simulink model "Test_SimFEAdapter"  (Simulink 7.5)
settings: Solver=FixedStepDiscrete  StartTime=0.0  StopTime=inf  FixedStep=samplePeriod  RelTol=1e-3  AbsTol=1e-6
PreLoadFcn:
  | initializeSimulation
InitFcn:
  | clear('all');
  | initializeSimulation;
values from neighbouring files (symbols this model uses):
  damperA = 0    [initializeSimulation.m]
  damperB = 0    [initializeSimulation.m]
  damperC = 0    [initializeSimulation.m]
  damperCanon = 1    [initializeSimulation.m]
  flowCanon = 3.85    [initializeSimulation.m]
  forceCanon = 1    [initializeSimulation.m]
  frictionA = 0    [initializeSimulation.m]
  frictionB = 0    [initializeSimulation.m]
  frictionC = 0    [initializeSimulation.m]
  gasConstant = 1.8    [initializeSimulation.m]
  lengthCanon = 1    [initializeSimulation.m]
  massA = 4.2    [initializeSimulation.m]
  massB = 2.5    [initializeSimulation.m]
  massC = 2.5    [initializeSimulation.m]
  massCanon = 0.002588    [initializeSimulation.m]
  maxDisplA = (stroke2A + endLength2A) * lengthCanon    (= 22)    [initializeSimulation.m]
  maxDisplB = (stroke2B + endLength2B) * lengthCanon    (= 42)    [initializeSimulation.m]
  maxDisplC = (stroke2C + endLength2C) * lengthCanon    (= 72)    [initializeSimulation.m]
  maxOilVolume = volume * (1 - (precharge/supplyPress)^(1/gasConstant))    (= 10.5071802963)    [initializeSimulation.m]
  maxVelocA = (maxFlowA * flowCanon / (area1A * areaCanon)) / velocCanon    [initializeSimulation.m]
  maxVelocB = (maxFlowB * flowCanon / (area1B * areaCanon)) / velocCanon    [initializeSimulation.m]
  maxVelocC = (maxFlowC * flowCanon / (area1C * areaCanon)) / velocCanon    [initializeSimulation.m]
  minDisplA = -(stroke1A + endLength1A) * lengthCanon    (= -22)    [initializeSimulation.m]
  minDisplB = -(stroke1B + endLength1B) * lengthCanon    (= -42)    [initializeSimulation.m]
  minDisplC = -(stroke1C + endLength1C) * lengthCanon    (= -72)    [initializeSimulation.m]
  minVelocA = -(maxFlowA * flowCanon / (area2A * areaCanon)) / velocCanon    [initializeSimulation.m]
  minVelocB = -(maxFlowB * flowCanon / (area2B * areaCanon)) / velocCanon    [initializeSimulation.m]
  minVelocC = -(maxFlowC * flowCanon / (area2C * areaCanon)) / velocCanon    [initializeSimulation.m]
  nAct = 8    [initializeSimulation.m]
  nAdcU = 12    [initializeSimulation.m]
  nDinp = 4    [initializeSimulation.m]
  nDout = 4    [initializeSimulation.m]
  nDucU = 8    [initializeSimulation.m]
  nEncU = 2    [initializeSimulation.m]
  precharge = 1000    [initializeSimulation.m]
  pumpFlow = 1e10    (= 10000000000)    [initializeSimulation.m]
  returnPress = 50    [initializeSimulation.m]
  staticForceA = 0    [initializeSimulation.m]
  staticForceB = 0    [initializeSimulation.m]
  staticForceC = 0    [initializeSimulation.m]
  supplyPress = 3000    [initializeSimulation.m]
  velocCanon = 1    [initializeSimulation.m]
  volume = accumVolume * accumNumber    (= 23)    [initializeSimulation.m]
  volumeCanon = 231    [initializeSimulation.m]
  yieldDisplA = 0.1    [initializeSimulation.m]
  yieldDisplB = 0.1    [initializeSimulation.m]
  yieldDisplC = 0.1    [initializeSimulation.m]
undefined symbols (not defined in the file or in its folder): DiscIntNeverNeededParam
(part 2 of 3)

== system Test_SimFEAdapter/model/ActuatorPayloadMdl/static channel #1/actuator/valve  model ==
  note: Note: "1" and "2" denote actuator
      | cylinders on either side of the
      | actuator piston.  With positive
      | valve drive, oil is ported into
      | cylinder 1, resulting in positive
      | displacement.
  note: Auxiliary diagnostic output vector:
      | 1:   valve opening
      | 2:   C1 pressure
      | 3:   C2 pressure
      | 4:   delta pressure
      | 5:   force
      | 6:   velocity
      | 7:   C1 flow
      | 8:   C2 flow
      | 9:   total flow
      | 10: kinematic flow
      | 11: compressibility flow
      | 12: leakage flow
  note: Parameter vector:
      | 1:   oil bulk modulus (force/displ^2)
      | 2:   servovalve delay (sec)
      | 3:   servovalve overlap
      | 4:   rated pressure (force/displ^2)
      | 5:   rated flow at rated pressure (displ^3/sec)
      | 6:   nominal flow at rated pressure (displ^3/sec)
      | 7:   actuator piston area 1 (displ^2)
      | 8:   actuator piston area 2 (displ^2)
      | 9:   actuator usable stroke 1 (displ)
      | 10: actuator usable stroke 2 (displ)
      | 11: actuator end cushion length 1 (displ)
      | 12: actuator end cushion length 2 (displ)
      | 13: actuator parasitic damping factor
      | 14: cross-chamber leakage factor (flow/press)
      | 15: ratio port openings according to area
      | 16: sample period (sec)
      |
      | Conversion factors used for converting
      | signals from external (user) to internal
      | (canonical) units:
      |
      | 17: displacement
      | 18: velocity
      | 19: force
      | 20: pressure
      | 21: flow
  cmd : Inport  OutDataType=sfix(16)  OutScaling=2^0
  displ : Inport  Port=2  OutDataType=sfix(16)  OutScaling=2^0
  veloc : Inport  Port=3  OutDataType=sfix(16)  OutScaling=2^0
  spl press : Inport  Port=4  OutDataType=sfix(16)  OutScaling=2^0
  rtn press : Inport  Port=5  OutDataType=sfix(16)  OutScaling=2^0
  abs : Abs  SaturateOnIntegerOverflow=on
  actuator : S-Function  FunctionName=actuator  Parameters=actParamsC  EnableBusSupport=off
  total flow sel : Selector  InputPortWidth=12  IndexOptions=Index vector (dialog)  Indices=9  OutputSizes=1
  force : Outport  OutDataType=sfix(16)  OutScaling=2^0
  flow : Outport  Port=2  OutDataType=sfix(16)  OutScaling=2^0
  wires:
  veloc/1 -> actuator/3
  displ/1 -> actuator/2
  actuator/1 -> force/1
  cmd/1 -> actuator/1
  rtn press/1 -> actuator/5
  spl press/1 -> actuator/4
  total flow sel/1 -> abs/1
  actuator/2 -> total flow sel/1
  abs/1 -> flow/1

== system Test_SimFEAdapter/model/ActuatorPayloadMdl/static channel #1/payload ==
  force : Inport  OutDataType=sfix(16)  OutScaling=2^0
  Sum : Sum  Inputs=+----  OutDataType=sfix(16)  OutScaling=2^0  SaturateOnIntegerOverflow=on  InputSameDT=on  OutDataTypeStr=Inherit: Same as first input
  damper : Gain  Gain=damperC*damperCanon  ParameterDataType=sfix(16)  ParameterScaling=2^0  OutDataType=sfix(16)  OutScaling=2^0  SaturateOnIntegerOverflow=on  OutDataTypeStr=Inherit: Same as input  ParamDataTypeStr=Inherit: Same as input
  div : Product  Inputs=*/  OutDataType=sfix(16)  OutScaling=2^0  SaturateOnIntegerOverflow=on  InputSameDT=on  OutDataTypeStr=Inherit: Same as first input
  double integrator : Subsystem
  friction : Subsystem  mask{friction=frictionC*forceCanon, yieldDispl=yieldDisplC*lengthCanon, hysteresis=0}
      mask prompts: friction "Sliding friction"; yieldDispl "Equiv. yield displacement (in)"; hysteresis "Hysteresis constant"
  mass : Constant  Value=massC*massCanon  OutDataType=sfix(16)  OutScaling=2^0
  static force : Constant  Value=staticForceC*forceCanon  OutDataType=sfix(16)  OutScaling=2^0
  term1 : Terminator
  unit dly : UnitDelay  SampleTime=-1
  unit dly1 : UnitDelay  SampleTime=-1
  veloc units : Gain  Gain=1/velocCanon  ParameterDataType=sfix(16)  ParameterScaling=2^0  OutDataType=sfix(16)  OutScaling=2^0  SaturateOnIntegerOverflow=on  OutDataTypeStr=Inherit: Same as input  ParamDataTypeStr=Inherit: Same as input
  displ : Outport  OutDataType=sfix(16)  OutScaling=2^0
  veloc : Outport  Port=2  OutDataType=sfix(16)  OutScaling=2^0
  tag scope: ch5a=global
  wires:
  friction/1(force) -> Sum/2  "friction force"
  veloc units/1 -> veloc/1
  Sum/1 -> div/1  "inertial force"
  force/1 -> Sum/1  "total force"
  mass/1 -> div/2
  double integrator/3(acc) -> term1/1
  div/1 -> double integrator/1(accel)
  double integrator/1(displ) -> displ/1, unit dly/1
  double integrator/2(veloc) -> veloc units/1, friction/1(veloc), unit dly1/1
  static force/1 -> Sum/5  "static force"
  damper/1 -> Sum/4  "damper force"
  unit dly1/1 -> damper/1
  [ch5b] -> Sum/3  "spring force"
  unit dly/1 -> [ch5a]

== system Test_SimFEAdapter/model/ActuatorPayloadMdl/static channel #2/actuator/valve  model ==
  note: Auxiliary diagnostic output vector:
      | 1:   valve opening
      | 2:   C1 pressure
      | 3:   C2 pressure
      | 4:   delta pressure
      | 5:   force
      | 6:   velocity
      | 7:   C1 flow
      | 8:   C2 flow
      | 9:   total flow
      | 10: kinematic flow
      | 11: compressibility flow
      | 12: leakage flow
  note: Note: "1" and "2" denote actuator
      | cylinders on either side of the
      | actuator piston.  With positive
      | valve drive, oil is ported into
      | cylinder 1, resulting in positive
      | displacement.
  note: Parameter vector:
      | 1:   oil bulk modulus (force/displ^2)
      | 2:   servovalve delay (sec)
      | 3:   servovalve overlap
      | 4:   rated pressure (force/displ^2)
      | 5:   rated flow at rated pressure (displ^3/sec)
      | 6:   nominal flow at rated pressure (displ^3/sec)
      | 7:   actuator piston area 1 (displ^2)
      | 8:   actuator piston area 2 (displ^2)
      | 9:   actuator usable stroke 1 (displ)
      | 10: actuator usable stroke 2 (displ)
      | 11: actuator end cushion length 1 (displ)
      | 12: actuator end cushion length 2 (displ)
      | 13: actuator parasitic damping factor
      | 14: cross-chamber leakage factor (flow/press)
      | 15: ratio port openings according to area
      | 16: sample period (sec)
      |
      | Conversion factors used for converting
      | signals from external (user) to internal
      | (canonical) units:
      |
      | 17: displacement
      | 18: velocity
      | 19: force
      | 20: pressure
      | 21: flow
  cmd : Inport  OutDataType=sfix(16)  OutScaling=2^0
  displ : Inport  Port=2  OutDataType=sfix(16)  OutScaling=2^0
  veloc : Inport  Port=3  OutDataType=sfix(16)  OutScaling=2^0
  spl press : Inport  Port=4  OutDataType=sfix(16)  OutScaling=2^0
  rtn press : Inport  Port=5  OutDataType=sfix(16)  OutScaling=2^0
  abs : Abs  SaturateOnIntegerOverflow=on
  actuator : S-Function  FunctionName=actuator  Parameters=actParamsC  EnableBusSupport=off
  total flow sel : Selector  InputPortWidth=12  IndexOptions=Index vector (dialog)  Indices=9  OutputSizes=1
  force : Outport  OutDataType=sfix(16)  OutScaling=2^0
  flow : Outport  Port=2  OutDataType=sfix(16)  OutScaling=2^0
  wires:
  abs/1 -> flow/1
  actuator/2 -> total flow sel/1
  total flow sel/1 -> abs/1
  spl press/1 -> actuator/4
  rtn press/1 -> actuator/5
  cmd/1 -> actuator/1
  actuator/1 -> force/1
  displ/1 -> actuator/2
  veloc/1 -> actuator/3

== system Test_SimFEAdapter/model/ActuatorPayloadMdl/static channel #2/payload ==
  force : Inport  OutDataType=sfix(16)  OutScaling=2^0
  Sum : Sum  Inputs=+----  OutDataType=sfix(16)  OutScaling=2^0  SaturateOnIntegerOverflow=on  InputSameDT=on  OutDataTypeStr=Inherit: Same as first input
  damper : Gain  Gain=damperC*damperCanon  ParameterDataType=sfix(16)  ParameterScaling=2^0  OutDataType=sfix(16)  OutScaling=2^0  SaturateOnIntegerOverflow=on  OutDataTypeStr=Inherit: Same as input  ParamDataTypeStr=Inherit: Same as input
  div : Product  Inputs=*/  OutDataType=sfix(16)  OutScaling=2^0  SaturateOnIntegerOverflow=on  InputSameDT=on  OutDataTypeStr=Inherit: Same as first input
  double integrator : Subsystem
  friction : Subsystem  mask{friction=frictionC*forceCanon, yieldDispl=yieldDisplC*lengthCanon, hysteresis=0}
      mask prompts: friction "Sliding friction"; yieldDispl "Equiv. yield displacement (in)"; hysteresis "Hysteresis constant"
  mass : Constant  Value=massC*massCanon  OutDataType=sfix(16)  OutScaling=2^0
  static force : Constant  Value=staticForceC*forceCanon  OutDataType=sfix(16)  OutScaling=2^0
  term1 : Terminator
  unit dly : UnitDelay  SampleTime=-1
  unit dly1 : UnitDelay  SampleTime=-1
  veloc units : Gain  Gain=1/velocCanon  ParameterDataType=sfix(16)  ParameterScaling=2^0  OutDataType=sfix(16)  OutScaling=2^0  SaturateOnIntegerOverflow=on  OutDataTypeStr=Inherit: Same as input  ParamDataTypeStr=Inherit: Same as input
  displ : Outport  OutDataType=sfix(16)  OutScaling=2^0
  veloc : Outport  Port=2  OutDataType=sfix(16)  OutScaling=2^0
  tag scope: ch6a=global
  wires:
  friction/1(force) -> Sum/2  "friction force"
  veloc units/1 -> veloc/1
  Sum/1 -> div/1  "inertial force"
  force/1 -> Sum/1  "total force"
  mass/1 -> div/2
  double integrator/3(acc) -> term1/1
  div/1 -> double integrator/1(accel)
  double integrator/1(displ) -> displ/1, unit dly/1
  double integrator/2(veloc) -> veloc units/1, friction/1(veloc), unit dly1/1
  static force/1 -> Sum/5  "static force"
  damper/1 -> Sum/4  "damper force"
  unit dly1/1 -> damper/1
  [ch6b] -> Sum/3  "spring force"
  unit dly/1 -> [ch6a]

== system Test_SimFEAdapter/model/ActuatorPayloadMdl/static channel #3/actuator/valve  model ==
  note: Note: "1" and "2" denote actuator
      | cylinders on either side of the
      | actuator piston.  With positive
      | valve drive, oil is ported into
      | cylinder 1, resulting in positive
      | displacement.
  note: Auxiliary diagnostic output vector:
      | 1:   valve opening
      | 2:   C1 pressure
      | 3:   C2 pressure
      | 4:   delta pressure
      | 5:   force
      | 6:   velocity
      | 7:   C1 flow
      | 8:   C2 flow
      | 9:   total flow
      | 10: kinematic flow
      | 11: compressibility flow
      | 12: leakage flow
  note: Parameter vector:
      | 1:   oil bulk modulus (force/displ^2)
      | 2:   servovalve delay (sec)
      | 3:   servovalve overlap
      | 4:   rated pressure (force/displ^2)
      | 5:   rated flow at rated pressure (displ^3/sec)
      | 6:   nominal flow at rated pressure (displ^3/sec)
      | 7:   actuator piston area 1 (displ^2)
      | 8:   actuator piston area 2 (displ^2)
      | 9:   actuator usable stroke 1 (displ)
      | 10: actuator usable stroke 2 (displ)
      | 11: actuator end cushion length 1 (displ)
      | 12: actuator end cushion length 2 (displ)
      | 13: actuator parasitic damping factor
      | 14: cross-chamber leakage factor (flow/press)
      | 15: ratio port openings according to area
      | 16: sample period (sec)
      |
      | Conversion factors used for converting
      | signals from external (user) to internal
      | (canonical) units:
      |
      | 17: displacement
      | 18: velocity
      | 19: force
      | 20: pressure
      | 21: flow
  cmd : Inport  OutDataType=sfix(16)  OutScaling=2^0
  displ : Inport  Port=2  OutDataType=sfix(16)  OutScaling=2^0
  veloc : Inport  Port=3  OutDataType=sfix(16)  OutScaling=2^0
  spl press : Inport  Port=4  OutDataType=sfix(16)  OutScaling=2^0
  rtn press : Inport  Port=5  OutDataType=sfix(16)  OutScaling=2^0
  abs : Abs  SaturateOnIntegerOverflow=on
  actuator : S-Function  FunctionName=actuator  Parameters=actParamsC  EnableBusSupport=off
  total flow sel : Selector  InputPortWidth=12  IndexOptions=Index vector (dialog)  Indices=9  OutputSizes=1
  force : Outport  OutDataType=sfix(16)  OutScaling=2^0
  flow : Outport  Port=2  OutDataType=sfix(16)  OutScaling=2^0
  wires:
  veloc/1 -> actuator/3
  displ/1 -> actuator/2
  actuator/1 -> force/1
  cmd/1 -> actuator/1
  rtn press/1 -> actuator/5
  spl press/1 -> actuator/4
  total flow sel/1 -> abs/1
  actuator/2 -> total flow sel/1
  abs/1 -> flow/1

== system Test_SimFEAdapter/model/ActuatorPayloadMdl/static channel #3/payload ==
  force : Inport  OutDataType=sfix(16)  OutScaling=2^0
  Sum : Sum  Inputs=+----  OutDataType=sfix(16)  OutScaling=2^0  SaturateOnIntegerOverflow=on  InputSameDT=on  OutDataTypeStr=Inherit: Same as first input
  damper : Gain  Gain=damperC*damperCanon  ParameterDataType=sfix(16)  ParameterScaling=2^0  OutDataType=sfix(16)  OutScaling=2^0  SaturateOnIntegerOverflow=on  OutDataTypeStr=Inherit: Same as input  ParamDataTypeStr=Inherit: Same as input
  div : Product  Inputs=*/  OutDataType=sfix(16)  OutScaling=2^0  SaturateOnIntegerOverflow=on  InputSameDT=on  OutDataTypeStr=Inherit: Same as first input
  double integrator : Subsystem
  friction : Subsystem  mask{friction=frictionC*forceCanon, yieldDispl=yieldDisplC*lengthCanon, hysteresis=0}
      mask prompts: friction "Sliding friction"; yieldDispl "Equiv. yield displacement (in)"; hysteresis "Hysteresis constant"
  mass : Constant  Value=massC*massCanon  OutDataType=sfix(16)  OutScaling=2^0
  static force : Constant  Value=staticForceC*forceCanon  OutDataType=sfix(16)  OutScaling=2^0
  term1 : Terminator
  unit dly : UnitDelay  SampleTime=-1
  unit dly1 : UnitDelay  SampleTime=-1
  veloc units : Gain  Gain=1/velocCanon  ParameterDataType=sfix(16)  ParameterScaling=2^0  OutDataType=sfix(16)  OutScaling=2^0  SaturateOnIntegerOverflow=on  OutDataTypeStr=Inherit: Same as input  ParamDataTypeStr=Inherit: Same as input
  displ : Outport  OutDataType=sfix(16)  OutScaling=2^0
  veloc : Outport  Port=2  OutDataType=sfix(16)  OutScaling=2^0
  tag scope: ch7a=global
  wires:
  friction/1(force) -> Sum/2  "friction force"
  veloc units/1 -> veloc/1
  Sum/1 -> div/1  "inertial force"
  force/1 -> Sum/1  "total force"
  mass/1 -> div/2
  double integrator/3(acc) -> term1/1
  div/1 -> double integrator/1(accel)
  double integrator/1(displ) -> displ/1, unit dly/1
  double integrator/2(veloc) -> veloc units/1, friction/1(veloc), unit dly1/1
  static force/1 -> Sum/5  "static force"
  damper/1 -> Sum/4  "damper force"
  unit dly1/1 -> damper/1
  [ch7b] -> Sum/3  "spring force"
  unit dly/1 -> [ch7a]

== system Test_SimFEAdapter/model/ActuatorPayloadMdl/static channel #4/actuator/valve  model ==
  note: Auxiliary diagnostic output vector:
      | 1:   valve opening
      | 2:   C1 pressure
      | 3:   C2 pressure
      | 4:   delta pressure
      | 5:   force
      | 6:   velocity
      | 7:   C1 flow
      | 8:   C2 flow
      | 9:   total flow
      | 10: kinematic flow
      | 11: compressibility flow
      | 12: leakage flow
  note: Note: "1" and "2" denote actuator
      | cylinders on either side of the
      | actuator piston.  With positive
      | valve drive, oil is ported into
      | cylinder 1, resulting in positive
      | displacement.
  note: Parameter vector:
      | 1:   oil bulk modulus (force/displ^2)
      | 2:   servovalve delay (sec)
      | 3:   servovalve overlap
      | 4:   rated pressure (force/displ^2)
      | 5:   rated flow at rated pressure (displ^3/sec)
      | 6:   nominal flow at rated pressure (displ^3/sec)
      | 7:   actuator piston area 1 (displ^2)
      | 8:   actuator piston area 2 (displ^2)
      | 9:   actuator usable stroke 1 (displ)
      | 10: actuator usable stroke 2 (displ)
      | 11: actuator end cushion length 1 (displ)
      | 12: actuator end cushion length 2 (displ)
      | 13: actuator parasitic damping factor
      | 14: cross-chamber leakage factor (flow/press)
      | 15: ratio port openings according to area
      | 16: sample period (sec)
      |
      | Conversion factors used for converting
      | signals from external (user) to internal
      | (canonical) units:
      |
      | 17: displacement
      | 18: velocity
      | 19: force
      | 20: pressure
      | 21: flow
  cmd : Inport  OutDataType=sfix(16)  OutScaling=2^0
  displ : Inport  Port=2  OutDataType=sfix(16)  OutScaling=2^0
  veloc : Inport  Port=3  OutDataType=sfix(16)  OutScaling=2^0
  spl press : Inport  Port=4  OutDataType=sfix(16)  OutScaling=2^0
  rtn press : Inport  Port=5  OutDataType=sfix(16)  OutScaling=2^0
  abs : Abs  SaturateOnIntegerOverflow=on
  actuator : S-Function  FunctionName=actuator  Parameters=actParamsC  EnableBusSupport=off
  total flow sel : Selector  InputPortWidth=12  IndexOptions=Index vector (dialog)  Indices=9  OutputSizes=1
  force : Outport  OutDataType=sfix(16)  OutScaling=2^0
  flow : Outport  Port=2  OutDataType=sfix(16)  OutScaling=2^0
  wires:
  abs/1 -> flow/1
  actuator/2 -> total flow sel/1
  total flow sel/1 -> abs/1
  spl press/1 -> actuator/4
  rtn press/1 -> actuator/5
  cmd/1 -> actuator/1
  actuator/1 -> force/1
  displ/1 -> actuator/2
  veloc/1 -> actuator/3

== system Test_SimFEAdapter/model/ActuatorPayloadMdl/static channel #4/payload ==
  force : Inport  OutDataType=sfix(16)  OutScaling=2^0
  Sum : Sum  Inputs=+----  OutDataType=sfix(16)  OutScaling=2^0  SaturateOnIntegerOverflow=on  InputSameDT=on  OutDataTypeStr=Inherit: Same as first input
  damper : Gain  Gain=damperC*damperCanon  ParameterDataType=sfix(16)  ParameterScaling=2^0  OutDataType=sfix(16)  OutScaling=2^0  SaturateOnIntegerOverflow=on  OutDataTypeStr=Inherit: Same as input  ParamDataTypeStr=Inherit: Same as input
  div : Product  Inputs=*/  OutDataType=sfix(16)  OutScaling=2^0  SaturateOnIntegerOverflow=on  InputSameDT=on  OutDataTypeStr=Inherit: Same as first input
  double integrator : Subsystem
  friction : Subsystem  mask{friction=frictionC*forceCanon, yieldDispl=yieldDisplC*lengthCanon, hysteresis=0}
      mask prompts: friction "Sliding friction"; yieldDispl "Equiv. yield displacement (in)"; hysteresis "Hysteresis constant"
  mass : Constant  Value=massC*massCanon  OutDataType=sfix(16)  OutScaling=2^0
  static force : Constant  Value=staticForceC*forceCanon  OutDataType=sfix(16)  OutScaling=2^0
  term1 : Terminator
  unit dly : UnitDelay  SampleTime=-1
  unit dly1 : UnitDelay  SampleTime=-1
  veloc units : Gain  Gain=1/velocCanon  ParameterDataType=sfix(16)  ParameterScaling=2^0  OutDataType=sfix(16)  OutScaling=2^0  SaturateOnIntegerOverflow=on  OutDataTypeStr=Inherit: Same as input  ParamDataTypeStr=Inherit: Same as input
  displ : Outport  OutDataType=sfix(16)  OutScaling=2^0
  veloc : Outport  Port=2  OutDataType=sfix(16)  OutScaling=2^0
  tag scope: ch8a=global
  wires:
  friction/1(force) -> Sum/2  "friction force"
  veloc units/1 -> veloc/1
  Sum/1 -> div/1  "inertial force"
  force/1 -> Sum/1  "total force"
  mass/1 -> div/2
  double integrator/3(acc) -> term1/1
  div/1 -> double integrator/1(accel)
  double integrator/1(displ) -> displ/1, unit dly/1
  double integrator/2(veloc) -> veloc units/1, friction/1(veloc), unit dly1/1
  static force/1 -> Sum/5  "static force"
  damper/1 -> Sum/4  "damper force"
  unit dly1/1 -> damper/1
  [ch8b] -> Sum/3  "spring force"
  unit dly/1 -> [ch8a]

== system Test_SimFEAdapter/model/ActuatorPayloadMdl/dynamic long channel #1/payload/double integrator ==
  accel : Inport
  displ gen : DiscreteIntegrator  IntegratorMethod=Integration: Backward Euler  SampleTime=-1  OutDataType=sfix(16)  OutScaling=2^0  LimitOutput=on  UpperSaturationLimit=maxDisplB  LowerSaturationLimit=minDisplB  ShowSaturationPort=on  ICPrevOutput=DiscIntNeverNeededParam  ICPrevScaledInput=DiscIntNeverNeededParam
  veloc gen : Subsystem  mask{maxVeloc=maxVelocB*velocCanon, minVeloc=minVelocB*velocCanon, maxDispl=maxDisplB, minDispl=minDisplB}
      mask prompts: maxVeloc "Max velocity"; minVeloc "Min velocity"; maxDispl "Max displacement"; minDispl "Min displacement"
  displ : Outport
  veloc : Outport  Port=2
  acc : Outport  Port=3
  wires:
  displ gen/2 -> veloc gen/3(reset)
  displ gen/1 -> displ/1, veloc gen/2(displ)
  veloc gen/1(veloc) -> displ gen/1, veloc/1
  accel/1 -> veloc gen/1(accel), acc/1

== system Test_SimFEAdapter/model/ActuatorPayloadMdl/dynamic long channel #1/payload/friction ==
  veloc : Inport  OutDataType=sfix(16)  OutScaling=2^0
  1-beta : Gain  Gain=1-hysteresis  ParameterDataType=sfix(16)  ParameterScaling=2^0  OutDataType=sfix(16)  OutScaling=2^0  SaturateOnIntegerOverflow=on  OutDataTypeStr=Inherit: Same as input  ParamDataTypeStr=Inherit: Same as input
  Sign : Signum
  Sum : Sum  Inputs=|++  OutDataType=sfix(16)  OutScaling=2^0  SaturateOnIntegerOverflow=on
  Sum1 : Sum  Inputs=|+-  OutDataType=sfix(16)  OutScaling=2^0  SaturateOnIntegerOverflow=on
  beta : Constant  Value=hysteresis  OutDataType=sfix(16)  OutScaling=2^0
  integrator : DiscreteIntegrator  SampleTime=-1  OutDataType=sfix(16)  OutScaling=2^0  LimitOutput=on  UpperSaturationLimit=1  LowerSaturationLimit=-1  ICPrevOutput=DiscIntNeverNeededParam  ICPrevScaledInput=DiscIntNeverNeededParam
  one : Constant  OutDataType=sfix(16)  OutScaling=2^0
  prod1 : Product  OutDataType=sfix(16)  OutScaling=2^0  SaturateOnIntegerOverflow=on  InputSameDT=on  OutDataTypeStr=Inherit: Same as first input
  prod2 : Product  OutDataType=sfix(16)  OutScaling=2^0  SaturateOnIntegerOverflow=on  InputSameDT=on  OutDataTypeStr=Inherit: Same as first input
  prod3 : Product  Inputs=3  OutDataType=sfix(16)  OutScaling=2^0  SaturateOnIntegerOverflow=on  InputSameDT=on  OutDataTypeStr=Inherit: Same as first input
  prod4 : Product  OutDataType=sfix(16)  OutScaling=2^0  SaturateOnIntegerOverflow=on  InputSameDT=on  OutDataTypeStr=Inherit: Same as first input
  sliding friction : Constant  Value=friction  OutDataType=sfix(16)  OutScaling=2^0
  y inv : Gain  Gain=1/max(eps, yieldDispl)  ParameterDataType=sfix(16)  ParameterScaling=2^0  OutDataType=sfix(16)  OutScaling=2^0  SaturateOnIntegerOverflow=on  OutDataTypeStr=Inherit: Same as input  ParamDataTypeStr=Inherit: Same as input
  force : Outport  OutDataType=sfix(16)  OutScaling=2^0
  wires:
  sliding friction/1 -> prod1/1
  prod1/1 -> force/1
  veloc/1 -> prod4/2, prod2/2
  prod4/1 -> Sign/1
  Sign/1 -> 1-beta/1
  1-beta/1 -> Sum/2
  beta/1 -> Sum/1
  Sum/1 -> prod3/3
  one/1 -> Sum1/1
  prod3/1 -> Sum1/2
  Sum1/1 -> prod2/1
  prod2/1 -> y inv/1
  y inv/1 -> integrator/1
  integrator/1 -> prod1/2, prod4/1, prod3/1, prod3/2  "zee"

== system Test_SimFEAdapter/model/ActuatorPayloadMdl/dynamic long channel #2/payload/double integrator ==
  accel : Inport
  displ gen : DiscreteIntegrator  IntegratorMethod=Integration: Backward Euler  SampleTime=-1  OutDataType=sfix(16)  OutScaling=2^0  LimitOutput=on  UpperSaturationLimit=maxDisplB  LowerSaturationLimit=minDisplB  ShowSaturationPort=on  ICPrevOutput=DiscIntNeverNeededParam  ICPrevScaledInput=DiscIntNeverNeededParam
  veloc gen : Subsystem  mask{maxVeloc=maxVelocB*velocCanon, minVeloc=minVelocB*velocCanon, maxDispl=maxDisplB, minDispl=minDisplB}
      mask prompts: maxVeloc "Max velocity"; minVeloc "Min velocity"; maxDispl "Max displacement"; minDispl "Min displacement"
  displ : Outport
  veloc : Outport  Port=2
  acc : Outport  Port=3
  wires:
  displ gen/2 -> veloc gen/3(reset)
  displ gen/1 -> displ/1, veloc gen/2(displ)
  veloc gen/1(veloc) -> displ gen/1, veloc/1
  accel/1 -> veloc gen/1(accel), acc/1

== system Test_SimFEAdapter/model/ActuatorPayloadMdl/dynamic long channel #2/payload/friction ==
  veloc : Inport  OutDataType=sfix(16)  OutScaling=2^0
  1-beta : Gain  Gain=1-hysteresis  ParameterDataType=sfix(16)  ParameterScaling=2^0  OutDataType=sfix(16)  OutScaling=2^0  SaturateOnIntegerOverflow=on  OutDataTypeStr=Inherit: Same as input  ParamDataTypeStr=Inherit: Same as input
  Sign : Signum
  Sum : Sum  Inputs=|++  OutDataType=sfix(16)  OutScaling=2^0  SaturateOnIntegerOverflow=on
  Sum1 : Sum  Inputs=|+-  OutDataType=sfix(16)  OutScaling=2^0  SaturateOnIntegerOverflow=on
  beta : Constant  Value=hysteresis  OutDataType=sfix(16)  OutScaling=2^0
  integrator : DiscreteIntegrator  SampleTime=-1  OutDataType=sfix(16)  OutScaling=2^0  LimitOutput=on  UpperSaturationLimit=1  LowerSaturationLimit=-1  ICPrevOutput=DiscIntNeverNeededParam  ICPrevScaledInput=DiscIntNeverNeededParam
  one : Constant  OutDataType=sfix(16)  OutScaling=2^0
  prod1 : Product  OutDataType=sfix(16)  OutScaling=2^0  SaturateOnIntegerOverflow=on  InputSameDT=on  OutDataTypeStr=Inherit: Same as first input
  prod2 : Product  OutDataType=sfix(16)  OutScaling=2^0  SaturateOnIntegerOverflow=on  InputSameDT=on  OutDataTypeStr=Inherit: Same as first input
  prod3 : Product  Inputs=3  OutDataType=sfix(16)  OutScaling=2^0  SaturateOnIntegerOverflow=on  InputSameDT=on  OutDataTypeStr=Inherit: Same as first input
  prod4 : Product  OutDataType=sfix(16)  OutScaling=2^0  SaturateOnIntegerOverflow=on  InputSameDT=on  OutDataTypeStr=Inherit: Same as first input
  sliding friction : Constant  Value=friction  OutDataType=sfix(16)  OutScaling=2^0
  y inv : Gain  Gain=1/max(eps, yieldDispl)  ParameterDataType=sfix(16)  ParameterScaling=2^0  OutDataType=sfix(16)  OutScaling=2^0  SaturateOnIntegerOverflow=on  OutDataTypeStr=Inherit: Same as input  ParamDataTypeStr=Inherit: Same as input
  force : Outport  OutDataType=sfix(16)  OutScaling=2^0
  wires:
  sliding friction/1 -> prod1/1
  prod1/1 -> force/1
  veloc/1 -> prod4/2, prod2/2
  prod4/1 -> Sign/1
  Sign/1 -> 1-beta/1
  1-beta/1 -> Sum/2
  beta/1 -> Sum/1
  Sum/1 -> prod3/3
  one/1 -> Sum1/1
  prod3/1 -> Sum1/2
  Sum1/1 -> prod2/1
  prod2/1 -> y inv/1
  y inv/1 -> integrator/1
  integrator/1 -> prod1/2, prod4/1, prod3/1, prod3/2  "zee"

== system Test_SimFEAdapter/model/ActuatorPayloadMdl/dynamic short channel #1/payload/double integrator ==
  accel : Inport
  displ gen : DiscreteIntegrator  IntegratorMethod=Integration: Backward Euler  SampleTime=-1  OutDataType=sfix(16)  OutScaling=2^0  LimitOutput=on  UpperSaturationLimit=maxDisplA  LowerSaturationLimit=minDisplA  ShowSaturationPort=on  ICPrevOutput=DiscIntNeverNeededParam  ICPrevScaledInput=DiscIntNeverNeededParam
  veloc gen : Subsystem  mask{maxVeloc=maxVelocA*velocCanon, minVeloc=minVelocA*velocCanon, maxDispl=maxDisplA, minDispl=minDisplA}
      mask prompts: maxVeloc "Max velocity"; minVeloc "Min velocity"; maxDispl "Max displacement"; minDispl "Min displacement"
  displ : Outport
  veloc : Outport  Port=2
  acc : Outport  Port=3
  wires:
  displ gen/2 -> veloc gen/3(reset)
  displ gen/1 -> displ/1, veloc gen/2(displ)
  veloc gen/1(veloc) -> displ gen/1, veloc/1
  accel/1 -> veloc gen/1(accel), acc/1

== system Test_SimFEAdapter/model/ActuatorPayloadMdl/dynamic short channel #1/payload/friction ==
  veloc : Inport  OutDataType=sfix(16)  OutScaling=2^0
  1-beta : Gain  Gain=1-hysteresis  ParameterDataType=sfix(16)  ParameterScaling=2^0  OutDataType=sfix(16)  OutScaling=2^0  SaturateOnIntegerOverflow=on  OutDataTypeStr=Inherit: Same as input  ParamDataTypeStr=Inherit: Same as input
  Sign : Signum
  Sum : Sum  Inputs=|++  OutDataType=sfix(16)  OutScaling=2^0  SaturateOnIntegerOverflow=on
  Sum1 : Sum  Inputs=|+-  OutDataType=sfix(16)  OutScaling=2^0  SaturateOnIntegerOverflow=on
  beta : Constant  Value=hysteresis  OutDataType=sfix(16)  OutScaling=2^0
  integrator : DiscreteIntegrator  SampleTime=-1  OutDataType=sfix(16)  OutScaling=2^0  LimitOutput=on  UpperSaturationLimit=1  LowerSaturationLimit=-1  ICPrevOutput=DiscIntNeverNeededParam  ICPrevScaledInput=DiscIntNeverNeededParam
  one : Constant  OutDataType=sfix(16)  OutScaling=2^0
  prod1 : Product  OutDataType=sfix(16)  OutScaling=2^0  SaturateOnIntegerOverflow=on  InputSameDT=on  OutDataTypeStr=Inherit: Same as first input
  prod2 : Product  OutDataType=sfix(16)  OutScaling=2^0  SaturateOnIntegerOverflow=on  InputSameDT=on  OutDataTypeStr=Inherit: Same as first input
  prod3 : Product  Inputs=3  OutDataType=sfix(16)  OutScaling=2^0  SaturateOnIntegerOverflow=on  InputSameDT=on  OutDataTypeStr=Inherit: Same as first input
  prod4 : Product  OutDataType=sfix(16)  OutScaling=2^0  SaturateOnIntegerOverflow=on  InputSameDT=on  OutDataTypeStr=Inherit: Same as first input
  sliding friction : Constant  Value=friction  OutDataType=sfix(16)  OutScaling=2^0
  y inv : Gain  Gain=1/max(eps, yieldDispl)  ParameterDataType=sfix(16)  ParameterScaling=2^0  OutDataType=sfix(16)  OutScaling=2^0  SaturateOnIntegerOverflow=on  OutDataTypeStr=Inherit: Same as input  ParamDataTypeStr=Inherit: Same as input
  force : Outport  OutDataType=sfix(16)  OutScaling=2^0
  wires:
  sliding friction/1 -> prod1/1
  prod1/1 -> force/1
  veloc/1 -> prod4/2, prod2/2
  prod4/1 -> Sign/1
  Sign/1 -> 1-beta/1
  1-beta/1 -> Sum/2
  beta/1 -> Sum/1
  Sum/1 -> prod3/3
  one/1 -> Sum1/1
  prod3/1 -> Sum1/2
  Sum1/1 -> prod2/1
  prod2/1 -> y inv/1
  y inv/1 -> integrator/1
  integrator/1 -> prod1/2, prod4/1, prod3/1, prod3/2  "zee"

== system Test_SimFEAdapter/model/ActuatorPayloadMdl/dynamic short channel #2/payload/double integrator ==
  accel : Inport
  displ gen : DiscreteIntegrator  IntegratorMethod=Integration: Backward Euler  SampleTime=-1  OutDataType=sfix(16)  OutScaling=2^0  LimitOutput=on  UpperSaturationLimit=maxDisplA  LowerSaturationLimit=minDisplA  ShowSaturationPort=on  ICPrevOutput=DiscIntNeverNeededParam  ICPrevScaledInput=DiscIntNeverNeededParam
  veloc gen : Subsystem  mask{maxVeloc=maxVelocA*velocCanon, minVeloc=minVelocA*velocCanon, maxDispl=maxDisplA, minDispl=minDisplA}
      mask prompts: maxVeloc "Max velocity"; minVeloc "Min velocity"; maxDispl "Max displacement"; minDispl "Min displacement"
  displ : Outport
  veloc : Outport  Port=2
  acc : Outport  Port=3
  wires:
  displ gen/2 -> veloc gen/3(reset)
  displ gen/1 -> displ/1, veloc gen/2(displ)
  veloc gen/1(veloc) -> displ gen/1, veloc/1
  accel/1 -> veloc gen/1(accel), acc/1

== system Test_SimFEAdapter/model/ActuatorPayloadMdl/dynamic short channel #2/payload/friction ==
  veloc : Inport  OutDataType=sfix(16)  OutScaling=2^0
  1-beta : Gain  Gain=1-hysteresis  ParameterDataType=sfix(16)  ParameterScaling=2^0  OutDataType=sfix(16)  OutScaling=2^0  SaturateOnIntegerOverflow=on  OutDataTypeStr=Inherit: Same as input  ParamDataTypeStr=Inherit: Same as input
  Sign : Signum
  Sum : Sum  Inputs=|++  OutDataType=sfix(16)  OutScaling=2^0  SaturateOnIntegerOverflow=on
  Sum1 : Sum  Inputs=|+-  OutDataType=sfix(16)  OutScaling=2^0  SaturateOnIntegerOverflow=on
  beta : Constant  Value=hysteresis  OutDataType=sfix(16)  OutScaling=2^0
  integrator : DiscreteIntegrator  SampleTime=-1  OutDataType=sfix(16)  OutScaling=2^0  LimitOutput=on  UpperSaturationLimit=1  LowerSaturationLimit=-1  ICPrevOutput=DiscIntNeverNeededParam  ICPrevScaledInput=DiscIntNeverNeededParam
  one : Constant  OutDataType=sfix(16)  OutScaling=2^0
  prod1 : Product  OutDataType=sfix(16)  OutScaling=2^0  SaturateOnIntegerOverflow=on  InputSameDT=on  OutDataTypeStr=Inherit: Same as first input
  prod2 : Product  OutDataType=sfix(16)  OutScaling=2^0  SaturateOnIntegerOverflow=on  InputSameDT=on  OutDataTypeStr=Inherit: Same as first input
  prod3 : Product  Inputs=3  OutDataType=sfix(16)  OutScaling=2^0  SaturateOnIntegerOverflow=on  InputSameDT=on  OutDataTypeStr=Inherit: Same as first input
  prod4 : Product  OutDataType=sfix(16)  OutScaling=2^0  SaturateOnIntegerOverflow=on  InputSameDT=on  OutDataTypeStr=Inherit: Same as first input
  sliding friction : Constant  Value=friction  OutDataType=sfix(16)  OutScaling=2^0
  y inv : Gain  Gain=1/max(eps, yieldDispl)  ParameterDataType=sfix(16)  ParameterScaling=2^0  OutDataType=sfix(16)  OutScaling=2^0  SaturateOnIntegerOverflow=on  OutDataTypeStr=Inherit: Same as input  ParamDataTypeStr=Inherit: Same as input
  force : Outport  OutDataType=sfix(16)  OutScaling=2^0
  wires:
  sliding friction/1 -> prod1/1
  prod1/1 -> force/1
  veloc/1 -> prod4/2, prod2/2
  prod4/1 -> Sign/1
  Sign/1 -> 1-beta/1
  1-beta/1 -> Sum/2
  beta/1 -> Sum/1
  Sum/1 -> prod3/3
  one/1 -> Sum1/1
  prod3/1 -> Sum1/2
  Sum1/1 -> prod2/1
  prod2/1 -> y inv/1
  y inv/1 -> integrator/1
  integrator/1 -> prod1/2, prod4/1, prod3/1, prod3/2  "zee"

== system Test_SimFEAdapter/model/ActuatorPayloadMdl/static channel #1/payload/double integrator ==
  accel : Inport
  displ gen : DiscreteIntegrator  IntegratorMethod=Integration: Backward Euler  SampleTime=-1  OutDataType=sfix(16)  OutScaling=2^0  LimitOutput=on  UpperSaturationLimit=maxDisplC  LowerSaturationLimit=minDisplC  ShowSaturationPort=on  ICPrevOutput=DiscIntNeverNeededParam  ICPrevScaledInput=DiscIntNeverNeededParam
  veloc gen : Subsystem  mask{maxVeloc=maxVelocC*velocCanon, minVeloc=minVelocC*velocCanon, maxDispl=maxDisplC, minDispl=minDisplC}
      mask prompts: maxVeloc "Max velocity"; minVeloc "Min velocity"; maxDispl "Max displacement"; minDispl "Min displacement"
  displ : Outport
  veloc : Outport  Port=2
  acc : Outport  Port=3
  wires:
  displ gen/2 -> veloc gen/3(reset)
  displ gen/1 -> displ/1, veloc gen/2(displ)
  veloc gen/1(veloc) -> displ gen/1, veloc/1
  accel/1 -> veloc gen/1(accel), acc/1

== system Test_SimFEAdapter/model/ActuatorPayloadMdl/static channel #1/payload/friction ==
  veloc : Inport  OutDataType=sfix(16)  OutScaling=2^0
  1-beta : Gain  Gain=1-hysteresis  ParameterDataType=sfix(16)  ParameterScaling=2^0  OutDataType=sfix(16)  OutScaling=2^0  SaturateOnIntegerOverflow=on  OutDataTypeStr=Inherit: Same as input  ParamDataTypeStr=Inherit: Same as input
  Sign : Signum
  Sum : Sum  Inputs=|++  OutDataType=sfix(16)  OutScaling=2^0  SaturateOnIntegerOverflow=on
  Sum1 : Sum  Inputs=|+-  OutDataType=sfix(16)  OutScaling=2^0  SaturateOnIntegerOverflow=on
  beta : Constant  Value=hysteresis  OutDataType=sfix(16)  OutScaling=2^0
  integrator : DiscreteIntegrator  SampleTime=-1  OutDataType=sfix(16)  OutScaling=2^0  LimitOutput=on  UpperSaturationLimit=1  LowerSaturationLimit=-1  ICPrevOutput=DiscIntNeverNeededParam  ICPrevScaledInput=DiscIntNeverNeededParam
  one : Constant  OutDataType=sfix(16)  OutScaling=2^0
  prod1 : Product  OutDataType=sfix(16)  OutScaling=2^0  SaturateOnIntegerOverflow=on  InputSameDT=on  OutDataTypeStr=Inherit: Same as first input
  prod2 : Product  OutDataType=sfix(16)  OutScaling=2^0  SaturateOnIntegerOverflow=on  InputSameDT=on  OutDataTypeStr=Inherit: Same as first input
  prod3 : Product  Inputs=3  OutDataType=sfix(16)  OutScaling=2^0  SaturateOnIntegerOverflow=on  InputSameDT=on  OutDataTypeStr=Inherit: Same as first input
  prod4 : Product  OutDataType=sfix(16)  OutScaling=2^0  SaturateOnIntegerOverflow=on  InputSameDT=on  OutDataTypeStr=Inherit: Same as first input
  sliding friction : Constant  Value=friction  OutDataType=sfix(16)  OutScaling=2^0
  y inv : Gain  Gain=1/max(eps, yieldDispl)  ParameterDataType=sfix(16)  ParameterScaling=2^0  OutDataType=sfix(16)  OutScaling=2^0  SaturateOnIntegerOverflow=on  OutDataTypeStr=Inherit: Same as input  ParamDataTypeStr=Inherit: Same as input
  force : Outport  OutDataType=sfix(16)  OutScaling=2^0
  wires:
  sliding friction/1 -> prod1/1
  prod1/1 -> force/1
  veloc/1 -> prod4/2, prod2/2
  prod4/1 -> Sign/1
  Sign/1 -> 1-beta/1
  1-beta/1 -> Sum/2
  beta/1 -> Sum/1
  Sum/1 -> prod3/3
  one/1 -> Sum1/1
  prod3/1 -> Sum1/2
  Sum1/1 -> prod2/1
  prod2/1 -> y inv/1
  y inv/1 -> integrator/1
  integrator/1 -> prod1/2, prod4/1, prod3/1, prod3/2  "zee"

== system Test_SimFEAdapter/model/ActuatorPayloadMdl/static channel #2/payload/double integrator ==
  accel : Inport
  displ gen : DiscreteIntegrator  IntegratorMethod=Integration: Backward Euler  SampleTime=-1  OutDataType=sfix(16)  OutScaling=2^0  LimitOutput=on  UpperSaturationLimit=maxDisplC  LowerSaturationLimit=minDisplC  ShowSaturationPort=on  ICPrevOutput=DiscIntNeverNeededParam  ICPrevScaledInput=DiscIntNeverNeededParam
  veloc gen : Subsystem  mask{maxVeloc=maxVelocC*velocCanon, minVeloc=minVelocC*velocCanon, maxDispl=maxDisplC, minDispl=minDisplC}
      mask prompts: maxVeloc "Max velocity"; minVeloc "Min velocity"; maxDispl "Max displacement"; minDispl "Min displacement"
  displ : Outport
  veloc : Outport  Port=2
  acc : Outport  Port=3
  wires:
  displ gen/2 -> veloc gen/3(reset)
  displ gen/1 -> displ/1, veloc gen/2(displ)
  veloc gen/1(veloc) -> displ gen/1, veloc/1
  accel/1 -> veloc gen/1(accel), acc/1

== system Test_SimFEAdapter/model/ActuatorPayloadMdl/static channel #2/payload/friction ==
  veloc : Inport  OutDataType=sfix(16)  OutScaling=2^0
  1-beta : Gain  Gain=1-hysteresis  ParameterDataType=sfix(16)  ParameterScaling=2^0  OutDataType=sfix(16)  OutScaling=2^0  SaturateOnIntegerOverflow=on  OutDataTypeStr=Inherit: Same as input  ParamDataTypeStr=Inherit: Same as input
  Sign : Signum
  Sum : Sum  Inputs=|++  OutDataType=sfix(16)  OutScaling=2^0  SaturateOnIntegerOverflow=on
  Sum1 : Sum  Inputs=|+-  OutDataType=sfix(16)  OutScaling=2^0  SaturateOnIntegerOverflow=on
  beta : Constant  Value=hysteresis  OutDataType=sfix(16)  OutScaling=2^0
  integrator : DiscreteIntegrator  SampleTime=-1  OutDataType=sfix(16)  OutScaling=2^0  LimitOutput=on  UpperSaturationLimit=1  LowerSaturationLimit=-1  ICPrevOutput=DiscIntNeverNeededParam  ICPrevScaledInput=DiscIntNeverNeededParam
  one : Constant  OutDataType=sfix(16)  OutScaling=2^0
  prod1 : Product  OutDataType=sfix(16)  OutScaling=2^0  SaturateOnIntegerOverflow=on  InputSameDT=on  OutDataTypeStr=Inherit: Same as first input
  prod2 : Product  OutDataType=sfix(16)  OutScaling=2^0  SaturateOnIntegerOverflow=on  InputSameDT=on  OutDataTypeStr=Inherit: Same as first input
  prod3 : Product  Inputs=3  OutDataType=sfix(16)  OutScaling=2^0  SaturateOnIntegerOverflow=on  InputSameDT=on  OutDataTypeStr=Inherit: Same as first input
  prod4 : Product  OutDataType=sfix(16)  OutScaling=2^0  SaturateOnIntegerOverflow=on  InputSameDT=on  OutDataTypeStr=Inherit: Same as first input
  sliding friction : Constant  Value=friction  OutDataType=sfix(16)  OutScaling=2^0
  y inv : Gain  Gain=1/max(eps, yieldDispl)  ParameterDataType=sfix(16)  ParameterScaling=2^0  OutDataType=sfix(16)  OutScaling=2^0  SaturateOnIntegerOverflow=on  OutDataTypeStr=Inherit: Same as input  ParamDataTypeStr=Inherit: Same as input
  force : Outport  OutDataType=sfix(16)  OutScaling=2^0
  wires:
  sliding friction/1 -> prod1/1
  prod1/1 -> force/1
  veloc/1 -> prod4/2, prod2/2
  prod4/1 -> Sign/1
  Sign/1 -> 1-beta/1
  1-beta/1 -> Sum/2
  beta/1 -> Sum/1
  Sum/1 -> prod3/3
  one/1 -> Sum1/1
  prod3/1 -> Sum1/2
  Sum1/1 -> prod2/1
  prod2/1 -> y inv/1
  y inv/1 -> integrator/1
  integrator/1 -> prod1/2, prod4/1, prod3/1, prod3/2  "zee"

== system Test_SimFEAdapter/model/ActuatorPayloadMdl/static channel #3/payload/double integrator ==
  accel : Inport
  displ gen : DiscreteIntegrator  IntegratorMethod=Integration: Backward Euler  SampleTime=-1  OutDataType=sfix(16)  OutScaling=2^0  LimitOutput=on  UpperSaturationLimit=maxDisplC  LowerSaturationLimit=minDisplC  ShowSaturationPort=on  ICPrevOutput=DiscIntNeverNeededParam  ICPrevScaledInput=DiscIntNeverNeededParam
  veloc gen : Subsystem  mask{maxVeloc=maxVelocC*velocCanon, minVeloc=minVelocC*velocCanon, maxDispl=maxDisplC, minDispl=minDisplC}
      mask prompts: maxVeloc "Max velocity"; minVeloc "Min velocity"; maxDispl "Max displacement"; minDispl "Min displacement"
  displ : Outport
  veloc : Outport  Port=2
  acc : Outport  Port=3
  wires:
  displ gen/2 -> veloc gen/3(reset)
  displ gen/1 -> displ/1, veloc gen/2(displ)
  veloc gen/1(veloc) -> displ gen/1, veloc/1
  accel/1 -> veloc gen/1(accel), acc/1

== system Test_SimFEAdapter/model/ActuatorPayloadMdl/static channel #3/payload/friction ==
  veloc : Inport  OutDataType=sfix(16)  OutScaling=2^0
  1-beta : Gain  Gain=1-hysteresis  ParameterDataType=sfix(16)  ParameterScaling=2^0  OutDataType=sfix(16)  OutScaling=2^0  SaturateOnIntegerOverflow=on  OutDataTypeStr=Inherit: Same as input  ParamDataTypeStr=Inherit: Same as input
  Sign : Signum
  Sum : Sum  Inputs=|++  OutDataType=sfix(16)  OutScaling=2^0  SaturateOnIntegerOverflow=on
  Sum1 : Sum  Inputs=|+-  OutDataType=sfix(16)  OutScaling=2^0  SaturateOnIntegerOverflow=on
  beta : Constant  Value=hysteresis  OutDataType=sfix(16)  OutScaling=2^0
  integrator : DiscreteIntegrator  SampleTime=-1  OutDataType=sfix(16)  OutScaling=2^0  LimitOutput=on  UpperSaturationLimit=1  LowerSaturationLimit=-1  ICPrevOutput=DiscIntNeverNeededParam  ICPrevScaledInput=DiscIntNeverNeededParam
  one : Constant  OutDataType=sfix(16)  OutScaling=2^0
  prod1 : Product  OutDataType=sfix(16)  OutScaling=2^0  SaturateOnIntegerOverflow=on  InputSameDT=on  OutDataTypeStr=Inherit: Same as first input
  prod2 : Product  OutDataType=sfix(16)  OutScaling=2^0  SaturateOnIntegerOverflow=on  InputSameDT=on  OutDataTypeStr=Inherit: Same as first input
  prod3 : Product  Inputs=3  OutDataType=sfix(16)  OutScaling=2^0  SaturateOnIntegerOverflow=on  InputSameDT=on  OutDataTypeStr=Inherit: Same as first input
  prod4 : Product  OutDataType=sfix(16)  OutScaling=2^0  SaturateOnIntegerOverflow=on  InputSameDT=on  OutDataTypeStr=Inherit: Same as first input
  sliding friction : Constant  Value=friction  OutDataType=sfix(16)  OutScaling=2^0
  y inv : Gain  Gain=1/max(eps, yieldDispl)  ParameterDataType=sfix(16)  ParameterScaling=2^0  OutDataType=sfix(16)  OutScaling=2^0  SaturateOnIntegerOverflow=on  OutDataTypeStr=Inherit: Same as input  ParamDataTypeStr=Inherit: Same as input
  force : Outport  OutDataType=sfix(16)  OutScaling=2^0
  wires:
  sliding friction/1 -> prod1/1
  prod1/1 -> force/1
  veloc/1 -> prod4/2, prod2/2
  prod4/1 -> Sign/1
  Sign/1 -> 1-beta/1
  1-beta/1 -> Sum/2
  beta/1 -> Sum/1
  Sum/1 -> prod3/3
  one/1 -> Sum1/1
  prod3/1 -> Sum1/2
  Sum1/1 -> prod2/1
  prod2/1 -> y inv/1
  y inv/1 -> integrator/1
  integrator/1 -> prod1/2, prod4/1, prod3/1, prod3/2  "zee"

== system Test_SimFEAdapter/model/ActuatorPayloadMdl/static channel #4/payload/double integrator ==
  accel : Inport
  displ gen : DiscreteIntegrator  IntegratorMethod=Integration: Backward Euler  SampleTime=-1  OutDataType=sfix(16)  OutScaling=2^0  LimitOutput=on  UpperSaturationLimit=maxDisplC  LowerSaturationLimit=minDisplC  ShowSaturationPort=on  ICPrevOutput=DiscIntNeverNeededParam  ICPrevScaledInput=DiscIntNeverNeededParam
  veloc gen : Subsystem  mask{maxVeloc=maxVelocC*velocCanon, minVeloc=minVelocC*velocCanon, maxDispl=maxDisplC, minDispl=minDisplC}
      mask prompts: maxVeloc "Max velocity"; minVeloc "Min velocity"; maxDispl "Max displacement"; minDispl "Min displacement"
  displ : Outport
  veloc : Outport  Port=2
  acc : Outport  Port=3
  wires:
  displ gen/2 -> veloc gen/3(reset)
  displ gen/1 -> displ/1, veloc gen/2(displ)
  veloc gen/1(veloc) -> displ gen/1, veloc/1
  accel/1 -> veloc gen/1(accel), acc/1

== system Test_SimFEAdapter/model/ActuatorPayloadMdl/static channel #4/payload/friction ==
  veloc : Inport  OutDataType=sfix(16)  OutScaling=2^0
  1-beta : Gain  Gain=1-hysteresis  ParameterDataType=sfix(16)  ParameterScaling=2^0  OutDataType=sfix(16)  OutScaling=2^0  SaturateOnIntegerOverflow=on  OutDataTypeStr=Inherit: Same as input  ParamDataTypeStr=Inherit: Same as input
  Sign : Signum
  Sum : Sum  Inputs=|++  OutDataType=sfix(16)  OutScaling=2^0  SaturateOnIntegerOverflow=on
  Sum1 : Sum  Inputs=|+-  OutDataType=sfix(16)  OutScaling=2^0  SaturateOnIntegerOverflow=on
  beta : Constant  Value=hysteresis  OutDataType=sfix(16)  OutScaling=2^0
  integrator : DiscreteIntegrator  SampleTime=-1  OutDataType=sfix(16)  OutScaling=2^0  LimitOutput=on  UpperSaturationLimit=1  LowerSaturationLimit=-1  ICPrevOutput=DiscIntNeverNeededParam  ICPrevScaledInput=DiscIntNeverNeededParam
  one : Constant  OutDataType=sfix(16)  OutScaling=2^0
  prod1 : Product  OutDataType=sfix(16)  OutScaling=2^0  SaturateOnIntegerOverflow=on  InputSameDT=on  OutDataTypeStr=Inherit: Same as first input
  prod2 : Product  OutDataType=sfix(16)  OutScaling=2^0  SaturateOnIntegerOverflow=on  InputSameDT=on  OutDataTypeStr=Inherit: Same as first input
  prod3 : Product  Inputs=3  OutDataType=sfix(16)  OutScaling=2^0  SaturateOnIntegerOverflow=on  InputSameDT=on  OutDataTypeStr=Inherit: Same as first input
  prod4 : Product  OutDataType=sfix(16)  OutScaling=2^0  SaturateOnIntegerOverflow=on  InputSameDT=on  OutDataTypeStr=Inherit: Same as first input
  sliding friction : Constant  Value=friction  OutDataType=sfix(16)  OutScaling=2^0
  y inv : Gain  Gain=1/max(eps, yieldDispl)  ParameterDataType=sfix(16)  ParameterScaling=2^0  OutDataType=sfix(16)  OutScaling=2^0  SaturateOnIntegerOverflow=on  OutDataTypeStr=Inherit: Same as input  ParamDataTypeStr=Inherit: Same as input
  force : Outport  OutDataType=sfix(16)  OutScaling=2^0
  wires:
  sliding friction/1 -> prod1/1
  prod1/1 -> force/1
  veloc/1 -> prod4/2, prod2/2
  prod4/1 -> Sign/1
  Sign/1 -> 1-beta/1
  1-beta/1 -> Sum/2
  beta/1 -> Sum/1
  Sum/1 -> prod3/3
  one/1 -> Sum1/1
  prod3/1 -> Sum1/2
  Sum1/1 -> prod2/1
  prod2/1 -> y inv/1
  y inv/1 -> integrator/1
  integrator/1 -> prod1/2, prod4/1, prod3/1, prod3/2  "zee"

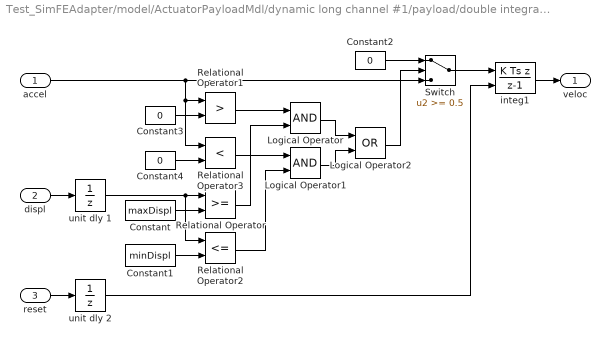
== system Test_SimFEAdapter/model/ActuatorPayloadMdl/dynamic long channel #1/payload/double integrator/veloc gen ==
  accel : Inport  OutDataType=sfix(16)  OutScaling=2^0
  displ : Inport  Port=2  OutDataType=sfix(16)  OutScaling=2^0
  reset : Inport  Port=3  OutDataType=sfix(16)  OutScaling=2^0
  Constant : Constant  Value=maxDispl  OutDataType=sfix(16)  OutScaling=2^0
  Constant1 : Constant  Value=minDispl  OutDataType=sfix(16)  OutScaling=2^0
  Constant2 : Constant  Value=0  OutDataType=sfix(16)  OutScaling=2^0
  Constant3 : Constant  Value=0  OutDataType=sfix(16)  OutScaling=2^0
  Constant4 : Constant  Value=0  OutDataType=sfix(16)  OutScaling=2^0
  Logical Operator : Logic
  Logical Operator1 : Logic
  Logical Operator2 : Logic  Operator=OR
  Relational Operator : RelationalOperator  InputSameDT=on
  Relational Operator1 : RelationalOperator  Operator=>  InputSameDT=on
  Relational Operator2 : RelationalOperator  Operator=<=  InputSameDT=on
  Relational Operator3 : RelationalOperator  Operator=<  InputSameDT=on
  Switch : Switch  Threshold=0.5  SaturateOnIntegerOverflow=on  InputSameDT=on
  integ1 : DiscreteIntegrator  IntegratorMethod=Integration: Backward Euler  ExternalReset=either  SampleTime=-1  OutDataType=sfix(16)  OutScaling=2^0  LimitOutput=on  UpperSaturationLimit=maxVeloc  LowerSaturationLimit=minVeloc  ICPrevOutput=DiscIntNeverNeededParam  ICPrevScaledInput=DiscIntNeverNeededParam
  unit dly 1 : UnitDelay  SampleTime=-1
  unit dly 2 : UnitDelay  SampleTime=-1
  veloc : Outport  OutDataType=sfix(16)  OutScaling=2^0
  wires:
  unit dly 1/1 -> Relational Operator2/1, Relational Operator/1
  reset/1 -> unit dly 2/1
  displ/1 -> unit dly 1/1
  Logical Operator1/1 -> Logical Operator2/2
  unit dly 2/1 -> integ1/2
  Switch/1 -> integ1/1
  Logical Operator2/1 -> Switch/2
  Constant2/1 -> Switch/1
  Logical Operator/1 -> Logical Operator2/1
  Relational Operator3/1 -> Logical Operator1/1
  Constant4/1 -> Relational Operator3/2
  Relational Operator1/1 -> Logical Operator/1
  Constant3/1 -> Relational Operator1/2
  accel/1 -> Switch/3, Relational Operator1/1, Relational Operator3/1
  Constant1/1 -> Relational Operator2/2
  Relational Operator2/1 -> Logical Operator1/2
  Relational Operator/1 -> Logical Operator/2
  Constant/1 -> Relational Operator/2
  integ1/1 -> veloc/1
